simulink model "dyno"  (R2017a)
settings: Solver=FixedStepDiscrete  StartTime=0.0  StopTime=0.5  FixedStep=abs(Ts)  RelTol=1e-3
values from neighbouring files (symbols this model uses):
  Ts = 1    [dynorun.m]
undefined symbols (not defined in the file or in its folder): elvio_tag_from, Fmax, Fmin
libraries: elvio x16
settings Model: Creator=tstef  LastModifiedBy=elts2

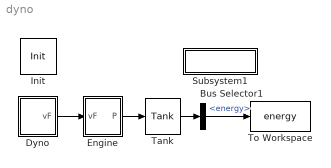
== system dyno ==
  Bus Selector1 : BusSelector  OutputSignals=energy
  Dyno : Subsystem  InitFcn=elvio_tag_from([1]);  mask(Dynamometer){speed=[100:20:500], load1=[5e3:1e3:55e3], FromTag1=Dyno1}
      mask prompts: speed "Speed [rad/s]:"; load1 "Load [W]:"; FromTag1 "Simulink:blkprm_prompts:FromGotoTag"
      mask help: This block is a virtual dynamometer. It injects a grid of speed and load points into a system, which is useful for getting an efficiency plot. Physical limits of the system are ignored, so it is possible to extrapolate.
      mask TypeOptions FromTag1: From/GotoTag
  Engine : Subsystem  AncestorBlock=elvio/Drive/Engine  InitFcn=|  mask(Loss Model){Tmax=110, Tmin=0, Tfrict=12, Ploss=1000, lossf=1.1, lossnorm=500e3, lossR=0.2, FromTag1=Engine1, GotoTag1=Dyno1}
      | elvio_tag_from([1]);
      | elvio_tag_goto([1]);
      mask prompts: Tmax "Max Torque:"; Tmin "Min Torque:"; Tfrict "Friction Torque (Nm):"; Ploss "Power Loss (W):"; lossf "Loss Factor (factor):"; lossnorm "Square Loss Normal (W):"; lossR "Slip Loss (rad/Nms):"; FromTag1 "Simulink:blkprm_prompts:FromGotoTag"; GotoTag1 "Simulink:blkprm_prompts:GotoTag"
      mask help: A simple parametric engine or motor model based on 5 loss models. See help for details.
      mask Help:
      | The five loss models are:
      |  * constant friction torque
      |  * constant power loss
      |  * constant efficiency loss
      |  * slip like loss (damping)
      |  * loss of square of the power, defined using the nomalized power where the loss equalls the full power
      | 
      | To create a model with twice the torque, the friction, power loss, and square loss have to doubled, and the slip damping has to be halved.
      | 
      | To create a model with twice the speed, the power loss, the slip damping, and the square power have to be doubled.
      mask TypeOptions FromTag1: From/GotoTag
      mask TypeOptions GotoTag1: Goto/GotoTag
  Init : elvio/Drive/Init  Ts0=1
  Subsystem1 : Subsystem
      settings: OpenFcn=|
      | efficiency = -load1./energy;
      | 
      | hold off
      | [c,h]=contour(speed,load1,efficiency);
      | clabel(c,h);
      | title('Efficiency coefficient');
      | xlabel('Speed in rad/s');
      | ylabel('Load in W');
      | hold on
      | plot(speed(1,:),Fmax(1,:).*speed(1,:));
      | hold off
      mask Display: disp('BSFC Plot')
  Tank : elvio/Drive/Tank  GotoTag1=Engine1
  "To Workspace " : ToWorkspace  VariableName=energy  SampleTime=-1
      settings: MaxDataPoints=1
  wires:
  Bus Selector1/1 -> "To Workspace "/1  "<energy>"
  Tank/1 -> Bus Selector1/1
  Dyno/1(vF) -> Engine/1(vF)
  Engine/1(P) -> Tank/1

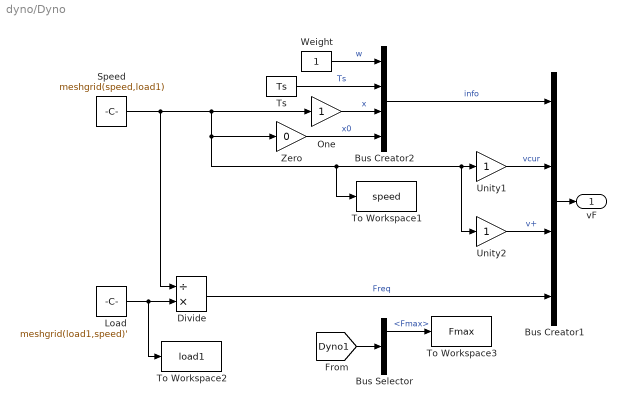
== system dyno/Dyno ==
  Bus Creator1 : BusCreator  Inputs=4
  Bus Creator2 : BusCreator  Inputs=4
  Bus Selector : BusSelector  OutputSignals=Fmax,Fmin
  Divide : Product  Inputs=/*
  Load : Constant  Value=meshgrid(load1,speed)'
  One : Gain
  Speed : Constant  Value=meshgrid(speed,load1)
  To Workspace1 : ToWorkspace  VariableName=speed  SampleTime=-1
      settings: MaxDataPoints=1
  To Workspace2 : ToWorkspace  VariableName=load1  SampleTime=-1
      settings: MaxDataPoints=1
  To Workspace3 : ToWorkspace  VariableName=Fmax  SampleTime=-1
      settings: MaxDataPoints=1
  Ts : Constant  Value=Ts
  Unity1 : Gain
  Unity2 : Gain
  Weight : Constant
  Zero : Gain  Gain=0
  vF : Outport
  wires:
  Speed/1 -> Divide/1, Zero/1, To Workspace1/1, Unity1/1, Unity2/1, One/1
  Unity1/1 -> Bus Creator1/2  "vcur"
  Bus Creator1/1 -> vF/1
  Divide/1 -> Bus Creator1/4  "Freq"
  Bus Creator2/1 -> Bus Creator1/1  "info"
  Unity2/1 -> Bus Creator1/3  "v+"
  [Dyno1] -> Bus Selector/1
  Load/1 -> To Workspace2/1, Divide/2
  One/1 -> Bus Creator2/3  "x"
  Ts/1 -> Bus Creator2/2  "Ts"
  Weight/1 -> Bus Creator2/1  "w"
  Zero/1 -> Bus Creator2/4  "x0"
  Bus Selector/1 -> To Workspace3/1  "<Fmax>"

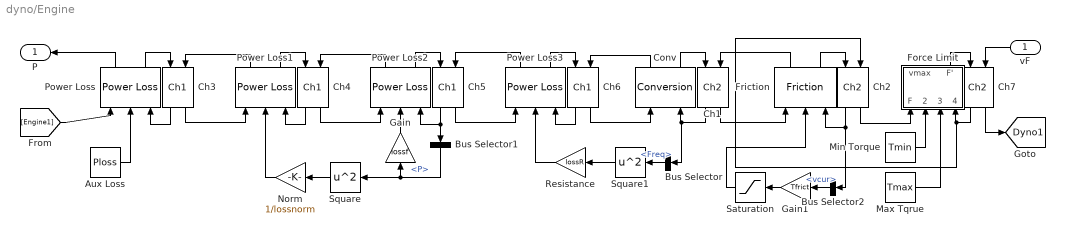
== system dyno/Engine ==
  vF : Inport
  Aux Loss : Constant  Value=Ploss
  Bus Selector : BusSelector  OutputSignals=Freq
  Bus Selector1 : BusSelector  OutputSignals=P
  Bus Selector2 : BusSelector  OutputSignals=vcur
  Ch1 : elvio/Basics/Ch2
  Ch2 : elvio/Basics/Ch2
  Ch{3..6} (4 alike) : elvio/Basics/Ch1
  Ch7 : elvio/Basics/Ch2
  Conv : elvio/Basics/Conversion
  Force Limit : Subsystem  AncestorBlock=elvio/Basics/Set Torque Limit
  Friction : elvio/Basics/Friction
  Gain : Gain  Gain=lossf
  Gain1 : Gain  Gain=Tfrict
  Max Tqrue : Constant  Value=Tmax
  Min Torque : Constant  Value=Tmin
  Norm : Gain  Gain=1/lossnorm
  Power Loss{,1..3} (4 alike) : elvio/Basics/Power Loss
  Resistance : Gain  Gain=lossR
  Saturation : Saturate  UpperLimit=Tfrict  LowerLimit=-Tfrict  ZeroCross=off
  Square : Math  Operator=square  SaturateOnIntegerOverflow=on
  Square1 : Math  Operator=square  SaturateOnIntegerOverflow=on
  P : Outport
  tag scope: Dyno1=global
  wires:
  Bus Selector2/1 -> Gain1/1  "<vcur>"
  Gain1/1 -> Saturation/1
  Min Torque/1 -> Force Limit/2(Min)
  Force Limit/2(F') -> Ch7/1
  vF/1 -> Ch7/2
  Ch7/2 -> [Dyno1]
  Resistance/1 -> Power Loss3/2
  Bus Selector/1 -> Square1/1  "<Freq>"
  Ch6/2 -> Conv/1
  Conv/1 -> Ch6/2
  Power Loss3/1 -> Ch5/2
  Power Loss3/2 -> Ch6/1
  Ch6/1 -> Power Loss3/3
  Ch5/2 -> Power Loss3/1
  Square1/1 -> Resistance/1
  Square/1 -> Norm/1
  Norm/1 -> Power Loss1/2
  Gain/1 -> Power Loss2/2
  Bus Selector1/1 -> Gain/1, Square/1  "<P>"
  Ch4/2 -> Power Loss2/1
  Ch5/1 -> Power Loss2/3, Bus Selector1/1
  Power Loss2/2 -> Ch5/1
  Power Loss2/1 -> Ch4/2
  Power Loss1/1 -> Ch3/2
  Power Loss1/2 -> Ch4/1
  Ch4/1 -> Power Loss1/3
  Ch3/2 -> Power Loss1/1
  [Engine1] -> Power Loss/1
  Ch1/1 -> Conv/2, Bus Selector/1
  Ch1/2 -> Friction/1
  Friction/1 -> Ch1/2
  Conv/2 -> Ch1/1
  Ch3/1 -> Power Loss/3
  Power Loss/2 -> Ch3/1
  Power Loss/1 -> P/1
  Ch2/2 -> Force Limit/1(F)
  Ch2/1 -> Friction/3, Bus Selector2/1
  Max Tqrue/1 -> Force Limit/3(Max)
  Aux Loss/1 -> Power Loss/2
  Friction/2 -> Ch2/1
  Saturation/1 -> Friction/2
  Ch7/1 -> Ch2/2, Force Limit/4(vreq)

== system dyno/Subsystem1 ==

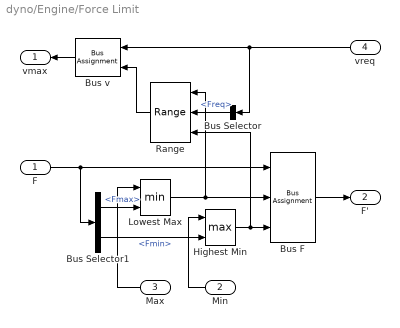
== system dyno/Engine/Force Limit ==
  F : Inport
  Min : Inport  Port=2
  Max : Inport  Port=3
  vreq : Inport  Port=4
  Bus Selector : BusSelector  OutputSignals=Freq
  Bus Selector1 : BusSelector  OutputSignals=Fmax,Fmin
  Bus F : BusAssignment  AssignedSignals=Fmax,Fmin
  Bus v : BusAssignment  AssignedSignals=Freq
  Highest Min : MinMax  Function=max  Inputs=2
  Lowest Max : MinMax  Inputs=2
  Range : elvio/Utilities/Range
  vmax : Outport
  F' : Outport  Port=2
  wires:
  Min/1 -> Highest Min/1
  Max/1 -> Lowest Max/1
  Bus Selector1/2 -> Highest Min/2  "<Fmin>"
  Bus Selector1/1 -> Lowest Max/2  "<Fmax>"
  Highest Min/1 -> Bus F/3, Range/3
  Lowest Max/1 -> Bus F/2, Range/1
  Bus F/1 -> F'/1
  Bus Selector/1 -> Range/2  "<Freq>"
  Range/1 -> Bus v/2
  vreq/1 -> Bus v/1, Bus Selector/1
  Bus v/1 -> vmax/1
  F/1 -> Bus F/1, Bus Selector1/1
